simulink model "scout"  (R2018a)
settings: Solver=FixedStepAuto  StartTime=0.0  StopTime=20  FixedStep=0.01  RelTol=1e-3
undefined symbols (not defined in the file): sigbuilder_block
libraries: simulink x4
settings Model: EnablePacing=on  Creator=U500304  LastModifiedBy=U500304
settings SolverCC: ZeroCrossAlgorithm=Adaptive
settings DataIOCC: SaveOutput=off  SaveTime=off
settings DebuggingCC: MaxConsecutiveZCsMsg=none

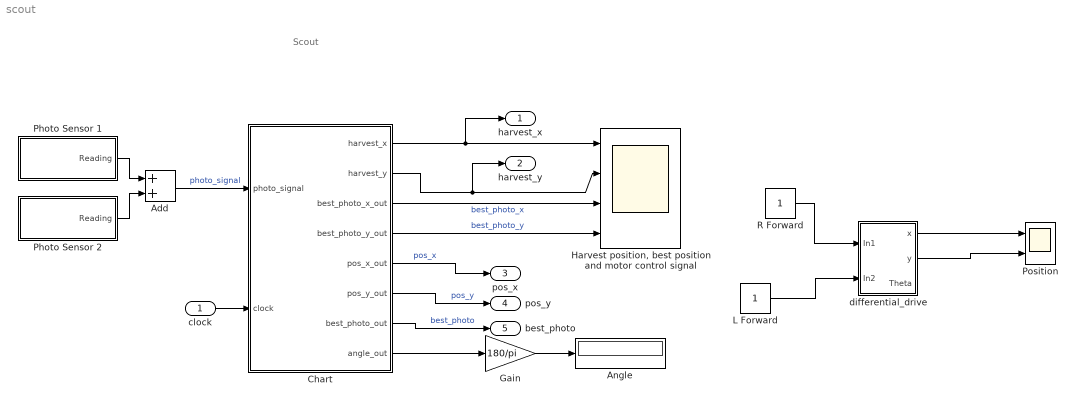
== system scout ==
  note: Scout
  clock : Inport  OutDataTypeStr=double  PortDimensions=1  SampleTime=0
  Add : Sum
  Angle : Display
  Chart : Stateflow chart  TreatAsAtomicUnit=on
  Gain : Gain  Gain=180/pi
  "Harvest position, best position and motor control signal" : Scope  NumInputPorts=4
  L Forward : Constant
  Photo Sensor 1 : Subsystem  Tag=STV Subsys  LoadFcn=sigbuilder_block('load');  StartFcn=sigbuilder_block('start');  StopFcn=sigbuilder_block('stop');  ClipboardFcn=sigbuilder_block('clipboard');  mask(Sigbuilder block){tuvar=[0:10]}
      mask help: Simulink:masks:SigbuilderBlock_MD
      mask init:
      | if ~strcmp(get_param(bdroot(gcbh),'SimulationStatus'),'stopped') tuvar = sigbuilder_block('maskInit'); end
      settings: CopyFcn=sigbuilder_block('copy');  DeleteFcn=sigbuilder_block('delete');  ModelCloseFcn=sigbuilder_block('modelClose');  PreSaveFcn=sigbuilder_block('preSave');  PauseFcn=sigbuilder_block('pause');  ContinueFcn=sigbuilder_block('continue');  NameChangeFcn=sigbuilder_block('namechange');  OpenFcn=sigbuilder_block('open',[5.4 30 1141.2 522.6 ]);  CloseFcn=sigbuilder_block('close');
      mask Display: plot(0, 0, 100, 100,[2, 2, 32, 32, 2], [68, 8, 8, 68, 68],[32, 2], [38, 38], [32, 19, 2],[53, 60, 44], [32, 17, 17, 2],[16, 16, 31, 31]);txt = getActiveGroup(gcbh);text(2, 100, txt,'verticalAlignment', 'top');
  Photo Sensor 2 : Subsystem  Tag=STV Subsys  LoadFcn=sigbuilder_block('load');  StartFcn=sigbuilder_block('start');  StopFcn=sigbuilder_block('stop');  ClipboardFcn=sigbuilder_block('clipboard');  mask(Sigbuilder block){tuvar=[0:10]}
      mask help: Simulink:masks:SigbuilderBlock_MD
      mask init:
      | if ~strcmp(get_param(bdroot(gcbh),'SimulationStatus'),'stopped') tuvar = sigbuilder_block('maskInit'); end
      settings: CopyFcn=sigbuilder_block('copy');  DeleteFcn=sigbuilder_block('delete');  ModelCloseFcn=sigbuilder_block('modelClose');  PreSaveFcn=sigbuilder_block('preSave');  PauseFcn=sigbuilder_block('pause');  ContinueFcn=sigbuilder_block('continue');  NameChangeFcn=sigbuilder_block('namechange');  OpenFcn=sigbuilder_block('open',[5.4 30 1141.2 522.6 ]);  CloseFcn=sigbuilder_block('close');
      mask Display: plot(0, 0, 100, 100,[2, 2, 32, 32, 2], [68, 8, 8, 68, 68],[32, 2], [38, 38], [32, 19, 2],[53, 60, 44], [32, 17, 17, 2],[16, 16, 31, 31]);txt = getActiveGroup(gcbh);text(2, 100, txt,'verticalAlignment', 'top');
  "Position " : Scope  NumInputPorts=2
  R Forward : Constant
  differential_drive : Subsystem
  harvest_x : Outport  OutDataTypeStr=double  PortDimensions=1  SampleTime=0
  harvest_y : Outport  Port=2  OutDataTypeStr=double  PortDimensions=1  SampleTime=0
  pos_x : Outport  Port=3  OutDataTypeStr=double  PortDimensions=1  SampleTime=0
  pos_y : Outport  Port=4  OutDataTypeStr=double  PortDimensions=1  SampleTime=0
  best_photo : Outport  Port=5  OutDataTypeStr=double  PortDimensions=1  SampleTime=0
  wires:
  Gain/1 -> Angle/1
  clock/1 -> Chart/2(clock)
  Add/1 -> Chart/1(photo_signal)  "photo_signal"
  Photo Sensor 2/1(Reading) -> Add/2
  Chart/6(pos_y_out) -> pos_y/1  "pos_y"
  Chart/4(best_photo_y_out) -> "Harvest position, best position and motor control signal"/4  "best_photo_y"
  Chart/8(angle_out) -> Gain/1
  Chart/3(best_photo_x_out) -> "Harvest position, best position and motor control signal"/3  "best_photo_x"
  Photo Sensor 1/1(Reading) -> Add/1
  Chart/1(harvest_x) -> "Harvest position, best position and motor control signal"/1, harvest_x/1
  Chart/2(harvest_y) -> harvest_y/1, "Harvest position, best position and motor control signal"/2
  Chart/5(pos_x_out) -> pos_x/1  "pos_x"
  Chart/7(best_photo_out) -> best_photo/1  "best_photo"
  R Forward/1 -> differential_drive/1(In1)
  L Forward/1 -> differential_drive/2(In2)
  differential_drive/1(x) -> "Position "/1
  differential_drive/2(y) -> "Position "/2

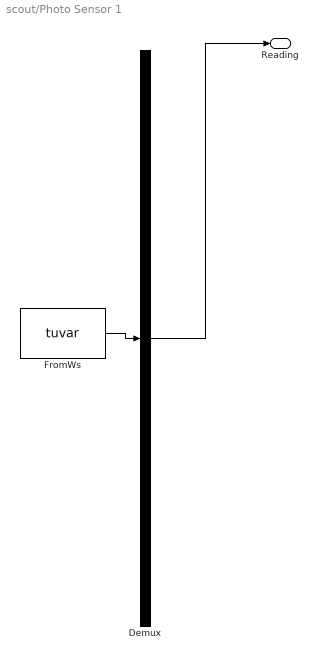
== system scout/Photo Sensor 1 ==
  Demux : Demux  Tag=STV Demux  Outputs=1
  FromWs : FromWorkspace  Tag=STV FromWs  VariableName=tuvar  SampleTime=0
      SigBuilderData=|
      | common.afterFinalStr = 'Extrapolate'
      | common.sampleTime = 0
      | dataSet.timeRange = [0 10]
      | dataSet.name = 'Photo Sensor'
      | sbobj.Groups.Name = 'Photo Sensor'
      | sbobj.Groups.Signals.Name = 'Reading'
      | sbobj.Groups.Signals.XData = [0 6 6 6.5 10]
      | sbobj.Groups.Signals.YData = [0 0 300 0 0]
  Reading : Outport  Tag=STV Outport
  wires:
  FromWs/1 -> Demux/1
  Demux/1 -> Reading/1

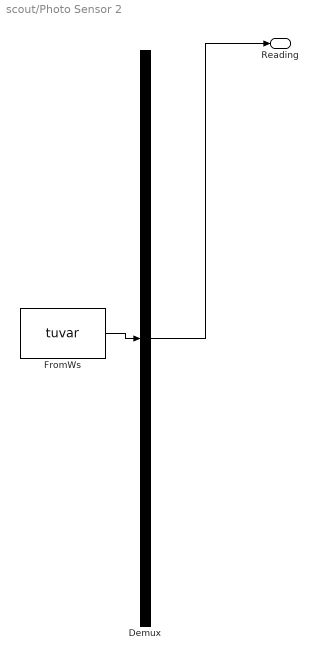
== system scout/Photo Sensor 2 ==
  Demux : Demux  Tag=STV Demux  Outputs=1
  FromWs : FromWorkspace  Tag=STV FromWs  VariableName=tuvar  SampleTime=0
      SigBuilderData=|
      | common.afterFinalStr = 'Extrapolate'
      | common.sampleTime = 0
      | dataSet.timeRange = [0 10]
      | dataSet.name = 'Photo Sensor'
      | sbobj.Groups.Name = 'Photo Sensor'
      | sbobj.Groups.Signals.Name = 'Reading'
      | sbobj.Groups.Signals.XData = [0 2 2 5 5 10]
      | sbobj.Groups.Signals.YData = [0 0 180 180 0 0]
  Reading : Outport  Tag=STV Outport
  wires:
  Demux/1 -> Reading/1
  FromWs/1 -> Demux/1

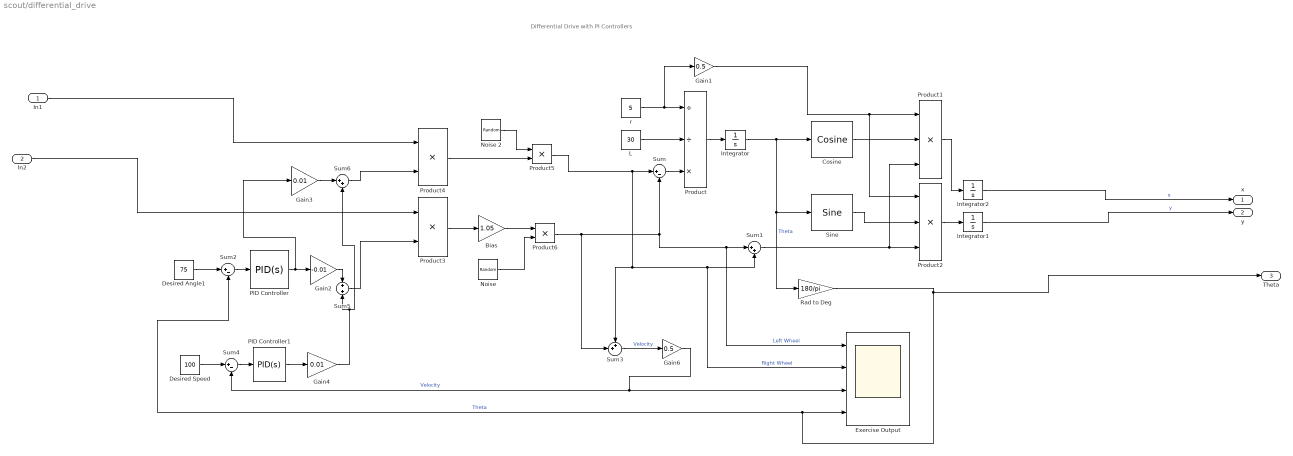
== system scout/differential_drive ==
  note: Differential Drive with PI Controllers
  In1 : Inport
  In2 : Inport  Port=2
  Bias : Gain  Gain=1.05
  Cosine : simulink/Lookup Tables/Cosine  Formula=cos(2*pi*u)  NumDataPoints=(2^5)+1  OutputWordLength=16  InternalRulePriority=Speed
      settings: SourceProductName=Simulink  SourceProductBaseCode=SL
  Desired Angle1 : Constant  Value=75
  Desired Speed : Constant  Value=100
  Exercise Output : Scope  NumInputPorts=4
  Gain1 : Gain  Gain=0.5
  Gain2 : Gain  Gain=-0.01
  Gain3 : Gain  Gain=0.01
  Gain4 : Gain  Gain=0.01
  Gain6 : Gain  Gain=0.5
  Integrator : Integrator
  Integrator1 : Integrator
  Integrator2 : Integrator
  L : Constant  Value=30
  Noise : UniformRandomNumber  Minimum=0.93  Maximum=1.07  Seed=637  SampleTime=0.1
  Noise 2 : UniformRandomNumber  Minimum=0.93  Maximum=1.07  Seed=521  SampleTime=0.1
  PID Controller : simulink/Continuous/PID Controller  Controller=PID  TimeDomain=Continuous-time  SampleTime=-1  IntegratorMethod=Forward Euler  FilterMethod=Forward Euler  Form=Parallel  UseFilter=on  ControllerParametersSource=internal  P=200  I=100  D=50  N=1  InitialConditionSource=internal  InitialConditionForIntegrator=0  InitialConditionForFilter=0  ExternalReset=none  LimitOutput=off  UpperSaturationLimit=100  LowerSaturationLimit=-100  LinearizeAsGain=on  AntiWindupMode=none  Kb=1  TrackingMode=off  Kt=1  PParamMin=[]  PParamMax=[]  IParamMin=[]  IParamMax=[]  DParamMin=[]  DParamMax=[]  NParamMin=[]  NParamMax=[]  KbParamMin=[]  KbParamMax=[]  KtParamMin=[]  KtParamMax=[]  POutMin=[]  POutMax=[]  IOutMin=[]  IOutMax=[]  DOutMin=[]  DOutMax=[]  NOutMin=[]  NOutMax=[]  KbOutMin=[]  KbOutMax=[]  KtOutMin=[]  KtOutMax=[]  IntegratorOutMin=[]  IntegratorOutMax=[]  FilterOutMin=[]  FilterOutMax=[]  SumOutMin=[]  SumOutMax=[]  SumI1OutMin=[]  SumI1OutMax=[]  SumI2OutMin=[]  SumI2OutMax=[]  SumI3OutMin=[]  SumI3OutMax=[]  SumDOutMin=[]  SumDOutMax=[]  SaturationOutMin=[]  SaturationOutMax=[]  IntegratorContinuousStateAttributes=''  IntegratorStateMustResolveToSignalObject=off  IntegratorRTWStateStorageClass=Auto  FilterContinuousStateAttributes=''  FilterStateMustResolveToSignalObject=off  FilterRTWStateStorageClass=Auto  DifferentiatorICPrevScaledInput=0  DifferentiatorOutMin=[]  DifferentiatorOutMax=[]  FilterDiffOutCoefMin=[]  FilterDiffOutCoefMax=[]  SumDenOutMin=[]  SumDenOutMax=[]  SumNumOutMin=[]  SumNumOutMax=[]  ReciprocalOutMin=[]  ReciprocalOutMax=[]  DivideOutMin=[]  DivideOutMax=[]  TunerSelectOption=Transfer Function Based (PID Tuner App)
  PID Controller1 : simulink/Continuous/PID Controller  Controller=PID  TimeDomain=Continuous-time  SampleTime=-1  IntegratorMethod=Forward Euler  FilterMethod=Forward Euler  Form=Parallel  UseFilter=on  ControllerParametersSource=internal  P=1  I=300  D=100  N=1  InitialConditionSource=internal  InitialConditionForIntegrator=0  InitialConditionForFilter=0  ExternalReset=none  LimitOutput=off  UpperSaturationLimit=inf  LowerSaturationLimit=-inf  LinearizeAsGain=on  AntiWindupMode=none  Kb=1  TrackingMode=off  Kt=1  PParamMin=[]  PParamMax=[]  IParamMin=[]  IParamMax=[]  DParamMin=[]  DParamMax=[]  NParamMin=[]  NParamMax=[]  KbParamMin=[]  KbParamMax=[]  KtParamMin=[]  KtParamMax=[]  POutMin=[]  POutMax=[]  IOutMin=[]  IOutMax=[]  DOutMin=[]  DOutMax=[]  NOutMin=[]  NOutMax=[]  KbOutMin=[]  KbOutMax=[]  KtOutMin=[]  KtOutMax=[]  IntegratorOutMin=[]  IntegratorOutMax=[]  FilterOutMin=[]  FilterOutMax=[]  SumOutMin=[]  SumOutMax=[]  SumI1OutMin=[]  SumI1OutMax=[]  SumI2OutMin=[]  SumI2OutMax=[]  SumI3OutMin=[]  SumI3OutMax=[]  SumDOutMin=[]  SumDOutMax=[]  SaturationOutMin=[]  SaturationOutMax=[]  IntegratorContinuousStateAttributes=''  IntegratorStateMustResolveToSignalObject=off  IntegratorRTWStateStorageClass=Auto  FilterContinuousStateAttributes=''  FilterStateMustResolveToSignalObject=off  FilterRTWStateStorageClass=Auto  DifferentiatorICPrevScaledInput=0  DifferentiatorOutMin=[]  DifferentiatorOutMax=[]  FilterDiffOutCoefMin=[]  FilterDiffOutCoefMax=[]  SumDenOutMin=[]  SumDenOutMax=[]  SumNumOutMin=[]  SumNumOutMax=[]  ReciprocalOutMin=[]  ReciprocalOutMax=[]  DivideOutMin=[]  DivideOutMax=[]  TunerSelectOption=Transfer Function Based (PID Tuner App)
  Product : Product  Inputs=//*
  Product1 : Product  Inputs=3
  Product2 : Product  Inputs=3
  Product{3..6} (4 alike) : Product
  Rad to Deg : Gain  Gain=180/pi
  Sine : simulink/Lookup Tables/Sine  Formula=sin(2*pi*u)  NumDataPoints=(2^5)+1  OutputWordLength=16  InternalRulePriority=Speed
      settings: SourceProductName=Simulink
  Sum : Sum  Inputs=|+-
  Sum1 : Sum  Inputs=|++
  Sum2 : Sum  Inputs=|+-
  Sum3 : Sum  Inputs=++|
  Sum4 : Sum  Inputs=|+-
  Sum5 : Sum
  Sum6 : Sum  Inputs=|++
  r : Constant  Value=5
  x : Outport
  y : Outport  Port=2
  Theta : Outport  Port=3
  wires:
  Product5/1 -> Sum/1, Sum3/1, Exercise Output/2, Sum1/2  "Right Wheel"
  Sum4/1 -> PID Controller1/1
  PID Controller1/1 -> Gain4/1
  Sum6/1 -> Product4/2
  Product4/1 -> Product5/2
  Gain6/1 -> Sum4/2, Exercise Output/3  "Velocity"
  L/1 -> Product/2
  Sum1/1 -> Product1/3, Product2/3
  Sum3/1 -> Gain6/1  "Velocity"
  In2/1 -> Product3/1
  Gain2/1 -> Sum5/1
  Sum5/1 -> Product3/2
  Gain4/1 -> Sum5/2, Sum6/2
  r/1 -> Gain1/1, Product/1
  PID Controller/1 -> Gain3/1, Gain2/1
  Rad to Deg/1 -> Theta/1, Sum2/2, Exercise Output/4  "Theta"
  Desired Angle1/1 -> Sum2/1
  Gain1/1 -> Product1/1, Product2/1
  Sine/1 -> Product2/2
  Product6/1 -> Sum/2, Exercise Output/1, Sum1/1, Sum3/2  "Left Wheel"
  Noise 2/1 -> Product5/1
  Bias/1 -> Product6/1
  Sum2/1 -> PID Controller/1
  Integrator/1 -> Rad to Deg/1, Sine/1, Cosine/1  "Theta"
  Gain3/1 -> Sum6/1
  Product/1 -> Integrator/1
  Product3/1 -> Bias/1
  Product2/1 -> Integrator1/1
  Cosine/1 -> Product1/2
  Desired Speed/1 -> Sum4/1
  In1/1 -> Product4/1
  Sum/1 -> Product/3
  Product1/1 -> Integrator2/1
  Noise/1 -> Product6/2
  Integrator1/1 -> y/1  "y"
  Integrator2/1 -> x/1  "x"

== stateflow chart scout/Chart ==
  settings: updateMethod=CONTINUOUS
  state Drive [parallel]
    settings: executionOrder=1
    state Move
      du:
      pos_x_dot = (r / 2) * (ul + ur) * cos(angle);
      pos_y_dot = (r / 2) * (ul + ur) * sin(angle);
      angle_dot = (r / L) * (ur - ul);
      pos_x_out = pos_x;
      pos_y_out = pos_y;
      angle_out = angle;
    note: Calculates robot's position based on wheel movements. Turns to 25 degrees left and drives straight on forever
    (default) -> Move : {
        | pos_x = 0;
        | pos_y = 0;
        | ul = 1;
        | ur = 1;
        | angle = 0;
        | turn = 0;
        | }
    Move -> Move [order 2] : [false]
        | {ul = 1; ur = -1; turn == 2;}
    Move -> Move [order 1] : [angle * 180/pi == 0 && turn == 0]
        | {ul = -1; ur = 1; turn = 1;}
    Move -> Move [order 3] : [angle * 180/pi  >= 25 && turn > 0]
        | {ul = 1; ur = 1; turn = 0}
  state Sense [parallel]
    settings: executionOrder=2
    state Dark
    state Light
      en, du:
      harvest_x = pos_x;
      harvest_y = pos_y;
    note: Senses the light and outputs harvest positions
    (default) -> Dark : {
        | best_photo = -1;
        | best_photo_x = -1;
        | best_photo_y = -1;
        | }
    Dark -> Light [order 1] : [photo_signal > 200]
    Dark -> Dark [order 2] : [photo_signal > best_photo]
        | {best_photo = photo_signal;
        | best_photo_x = pos_x;
        | best_photo_y = pos_y;}
    Light -> Dark [order 2] : [photo_signal <= 200]
    Light -> Light [order 1] : [photo_signal > best_photo]
        | {best_photo = photo_signal;
        | best_photo_x = pos_x;
        | best_photo_y = pos_y;}
  state Clock [parallel]
    settings: executionOrder=3
    state Seeking
      en:
      cycle_start = clock;
    state Report
      en:
      best_photo_out = best_photo;
      best_photo_x_out = best_photo_x;
      best_photo_y_out = best_photo_y;
    note: Updates the best harvest position
        | and light reading every 2 seconds
    (default) -> Seeking
    Report -> Seeking
    Seeking -> Report : [clock - cycle_start >= 2]
  data: photo_signal input; harvest_x output =-1; harvest_y output =-1; best_photo_x_out output =-1; best_photo_y_out output =-1; pos_x_out output; pos_y_out output; pos_x local; pos_y local; clock input; best_photo_out output =-1; best_photo local =0; best_photo_x local; best_photo_y local; cycle_start local; ur local double =1; ul local =1; angle local =0; r constant double =10; L constant double =100; angle_out output; turn local
  data pos_x settings: updateMethod=SF_CONTINUOUS_TIME_DATA
  data pos_y settings: updateMethod=SF_CONTINUOUS_TIME_DATA
  data angle settings: updateMethod=SF_CONTINUOUS_TIME_DATA
